simulink model "TrajectoryControl"  (R2020b)
settings: Solver=ode3  StartTime=0.0  StopTime=100.0  FixedStep=Ts  RelTol=1e-3
values from neighbouring files (symbols this model uses):
  obsx = 4    [Ejercicio1.m]    (also in Ejercicio2.m = 2.03)
  obsy = 0    [Ejercicio1.m]    (also in Ejercicio2.m = 1)
  th_0 = 0    [Ejercicio2.m]
  Ts = 100e-3    (= 0.1)    [Ejercicio1.m]    (also in Ejercicio2.m)
  x_0 = 0.02    [Ejercicio2.m]
  y_0 = 0    [Ejercicio2.m]
undefined symbols (not defined in the file or in its folder): DiscIntNeverNeededParam, sigbuilder_block
libraries: fuzblock x1, simulink x1
settings Model: Creator=patri  LastModifiedBy=Victor
settings DataIOCC: SaveOutput=off  ReturnWorkspaceOutputs=off

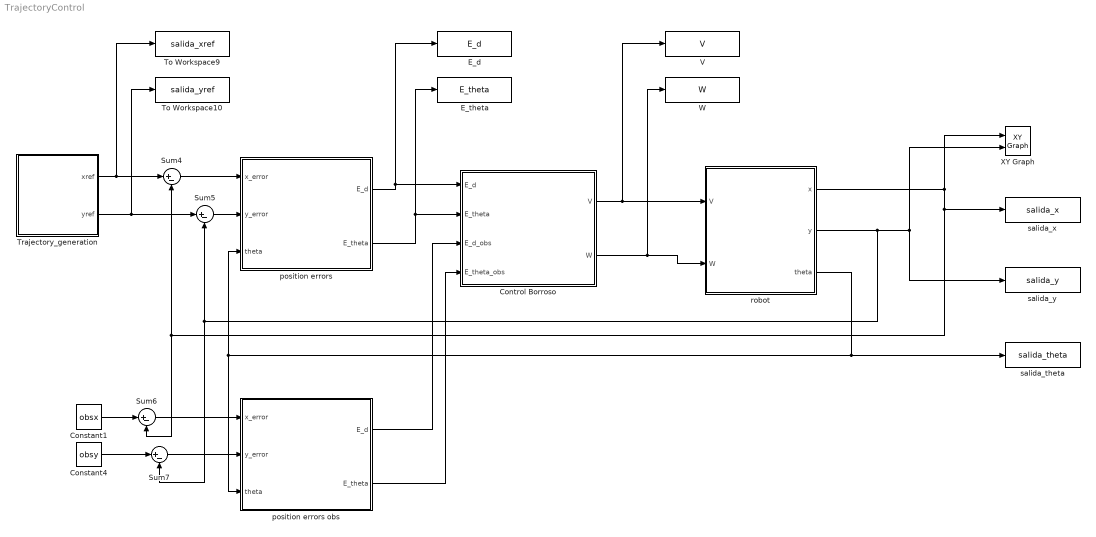
== system TrajectoryControl ==
  Constant1 : Constant  Value=obsx
  Constant4 : Constant  Value=obsy
  Control Borroso : Subsystem
  E_d : ToWorkspace  VariableName=E_d  SaveFormat=Structure With Time  SampleTime=-1
  E_theta : ToWorkspace  VariableName=E_theta  SaveFormat=Structure With Time  SampleTime=-1
  Sum{4..7} (4 alike) : Sum  Inputs=|+-
  To Workspace10 : ToWorkspace  VariableName=salida_yref  SaveFormat=Structure With Time  SampleTime=-1
  To Workspace9 : ToWorkspace  VariableName=salida_xref  SaveFormat=Structure With Time  SampleTime=-1
  Trajectory_generation : Subsystem
  V : ToWorkspace  VariableName=V  SaveFormat=Structure With Time  SampleTime=-1
  W : ToWorkspace  VariableName=W  SaveFormat=Structure With Time  SampleTime=-1
  XY Graph : simulink/Sinks/XY Graph  xmin=-10  xmax=10  ymin=-10  ymax=10  st=-1
  position errors : Subsystem
  position errors obs : Subsystem
  robot : Subsystem
  salida_theta : ToWorkspace  VariableName=salida_theta  SaveFormat=Structure With Time  SampleTime=-1
  salida_x : ToWorkspace  VariableName=salida_x  SaveFormat=Structure With Time  SampleTime=-1
  salida_y : ToWorkspace  VariableName=salida_y  SaveFormat=Structure With Time  SampleTime=-1
  wires:
  position errors obs/1(E_d) -> Control Borroso/3(E_d_obs)
  Trajectory_generation/1(xref) -> To Workspace9/1, Sum4/1
  Trajectory_generation/2(yref) -> To Workspace10/1, Sum5/1
  position errors/2(E_theta) -> Control Borroso/2(E_theta), E_theta/1
  Control Borroso/2("W ") -> robot/2(W), W/1
  Sum7/1 -> position errors obs/2(y_error)
  Constant4/1 -> Sum7/1
  position errors obs/2(E_theta) -> Control Borroso/4(E_theta_obs)
  Sum4/1 -> position errors/1(x_error)
  Constant1/1 -> Sum6/1
  Sum6/1 -> position errors obs/1(x_error)
  Sum5/1 -> position errors/2(y_error)
  robot/2(y) -> salida_y/1, XY Graph/2, Sum5/2, Sum7/2
  Control Borroso/1(V) -> V/1, robot/1(V)
  robot/1(x) -> salida_x/1, Sum4/2, Sum6/2, XY Graph/1
  position errors/1(E_d) -> Control Borroso/1("E_d "), E_d/1
  robot/3(theta) -> salida_theta/1, position errors obs/3(theta), position errors/3(theta)

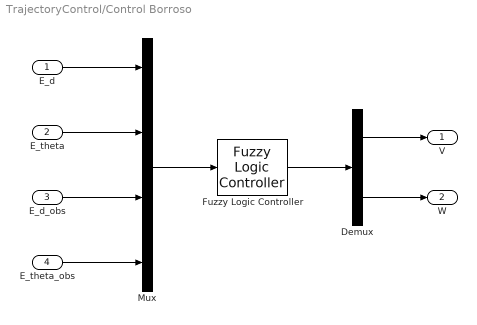
== system TrajectoryControl/Control Borroso ==
  "E_d " : Inport
  E_theta : Inport  Port=2
  E_d_obs : Inport  Port=3
  E_theta_obs : Inport  Port=4
  Demux : Demux  Outputs=2
  Fuzzy Logic Controller : fuzblock/Fuzzy Logic  Controller  FIS='ControlBorroso.fis'  OutputSampleNumber=101  DataType=double  FuzzifiedInputs=off  RuleFiringStrengths=off  RuleOutputs=off  AggregatedOutputs=off  SimulateUsing=Interpreted execution  OutOfRangeInputValueMessage=warning  NoRuleFiredMessage=warning  EmptyOutputFuzzySetMessage=warning
  Mux : Mux
  V : Outport  VectorParamsAs1DForOutWhenUnconnected=off
  "W " : Outport  Port=2  VectorParamsAs1DForOutWhenUnconnected=off
  wires:
  Mux/1 -> Fuzzy Logic Controller/1
  "E_d "/1 -> Mux/1
  Demux/1 -> V/1
  Demux/2 -> "W "/1
  E_theta/1 -> Mux/2
  E_d_obs/1 -> Mux/3
  E_theta_obs/1 -> Mux/4
  Fuzzy Logic Controller/1 -> Demux/1

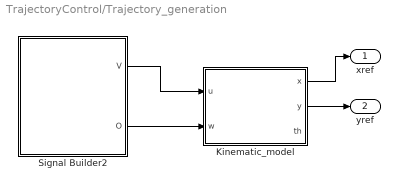
== system TrajectoryControl/Trajectory_generation ==
  Kinematic_model : Subsystem
  Signal Builder2 : Subsystem  Tag=STV Subsys  LoadFcn=sigbuilder_block('load');  StartFcn=sigbuilder_block('start');  StopFcn=sigbuilder_block('stop');  ClipboardFcn=sigbuilder_block('clipboard');  mask(Sigbuilder block){tuvar=[0:10]}
      mask help: Sigbuilder GUI
      mask init:
      | if ~strcmp(get_param(bdroot(gcbh),'SimulationStatus'),'stopped') tuvar = sigbuilder_block('maskInit'); end
      settings: CopyFcn=sigbuilder_block('copy');  DeleteFcn=sigbuilder_block('delete');  ModelCloseFcn=sigbuilder_block('modelClose');  PreSaveFcn=sigbuilder_block('preSave');  PauseFcn=sigbuilder_block('pause')  ContinueFcn=sigbuilder_block('continue')  NameChangeFcn=sigbuilder_block('namechange');  OpenFcn=sigbuilder_block('open',[60 45 534.4 467.25 ]);  CloseFcn=sigbuilder_block('close');
      mask Display: plot(0, 0, 100, 100,[2, 2, 32, 32, 2], [68, 8, 8, 68, 68],[32, 2], [38, 38], [32, 19, 2],[53, 60, 44], [32, 17, 17, 2],[16, 16, 31, 31]);txt = getActiveGroup(gcbh);text(2, 100, txt,'verticalAlignment', 'top');
  xref : Outport  VectorParamsAs1DForOutWhenUnconnected=off
  yref : Outport  Port=2  VectorParamsAs1DForOutWhenUnconnected=off
  wires:
  Kinematic_model/2(y) -> yref/1
  Kinematic_model/1(x) -> xref/1
  Signal Builder2/2(O) -> Kinematic_model/2(w)
  Signal Builder2/1(V) -> Kinematic_model/1(u)

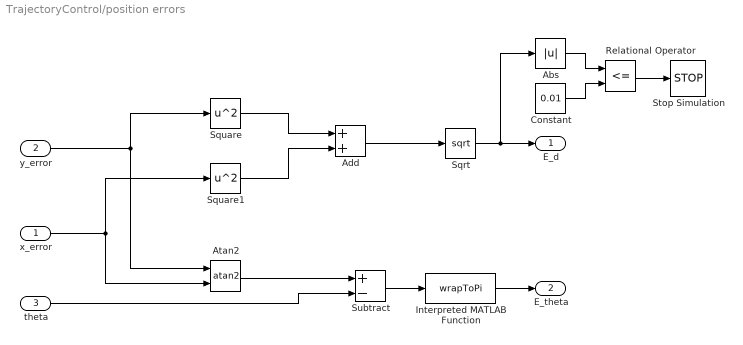
== system TrajectoryControl/position errors ==
  x_error : Inport
  y_error : Inport  Port=2
  theta : Inport  Port=3
  Abs : Abs
  Add : Sum
  Atan2 : Trigonometry  Operator=atan2
  Constant : Constant  Value=0.01
  Interpreted MATLAB Function : MATLABFcn  MATLABFcn=wrapToPi
  Relational Operator : RelationalOperator  Operator=<=  OutDataTypeStr=boolean  RndMeth=Simplest
  Sqrt : Sqrt  SaturateOnIntegerOverflow=on
  Square : Math  Operator=square  SignedPower=on  SaturateOnIntegerOverflow=on
  Square1 : Math  Operator=square  SignedPower=on  SaturateOnIntegerOverflow=on
  Stop Simulation : Stop
  Subtract : Sum  Inputs=+-  OutMin=[-3.14]  OutMax=[3.14]
  E_d : Outport  VectorParamsAs1DForOutWhenUnconnected=off
  E_theta : Outport  Port=2  OutMin=[-pi]  OutMax=[pi]  VectorParamsAs1DForOutWhenUnconnected=off
  wires:
  y_error/1 -> Atan2/1, Square/1
  x_error/1 -> Atan2/2, Square1/1
  Square/1 -> Add/1
  Square1/1 -> Add/2
  Add/1 -> Sqrt/1
  Sqrt/1 -> Abs/1, E_d/1
  Atan2/1 -> Subtract/1
  theta/1 -> Subtract/2
  Abs/1 -> Relational Operator/1
  Constant/1 -> Relational Operator/2
  Relational Operator/1 -> Stop Simulation/1
  Interpreted MATLAB Function/1 -> E_theta/1
  Subtract/1 -> Interpreted MATLAB Function/1

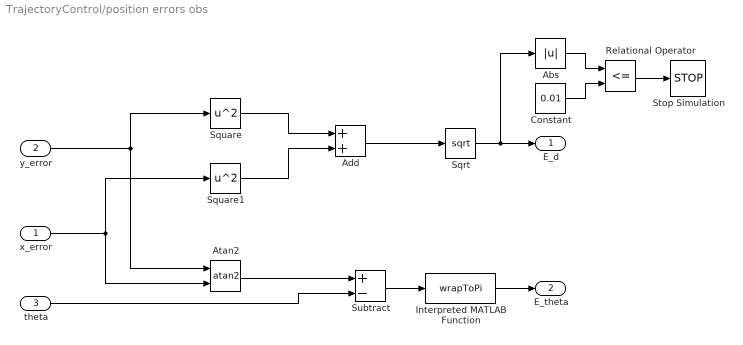
== system TrajectoryControl/position errors obs ==
  x_error : Inport
  y_error : Inport  Port=2
  theta : Inport  Port=3
  Abs : Abs
  Add : Sum
  Atan2 : Trigonometry  Operator=atan2
  Constant : Constant  Value=0.01
  Interpreted MATLAB Function : MATLABFcn  MATLABFcn=wrapToPi
  Relational Operator : RelationalOperator  Operator=<=  OutDataTypeStr=boolean  RndMeth=Simplest
  Sqrt : Sqrt  SaturateOnIntegerOverflow=on
  Square : Math  Operator=square  SignedPower=on  SaturateOnIntegerOverflow=on
  Square1 : Math  Operator=square  SignedPower=on  SaturateOnIntegerOverflow=on
  Stop Simulation : Stop
  Subtract : Sum  Inputs=+-
  E_d : Outport  VectorParamsAs1DForOutWhenUnconnected=off
  E_theta : Outport  Port=2  OutMin=[-pi]  OutMax=[pi]  VectorParamsAs1DForOutWhenUnconnected=off
  wires:
  y_error/1 -> Atan2/1, Square/1
  x_error/1 -> Atan2/2, Square1/1
  Square/1 -> Add/1
  Square1/1 -> Add/2
  Add/1 -> Sqrt/1
  Sqrt/1 -> Abs/1, E_d/1
  Atan2/1 -> Subtract/1
  theta/1 -> Subtract/2
  Abs/1 -> Relational Operator/1
  Constant/1 -> Relational Operator/2
  Relational Operator/1 -> Stop Simulation/1
  Subtract/1 -> Interpreted MATLAB Function/1
  Interpreted MATLAB Function/1 -> E_theta/1

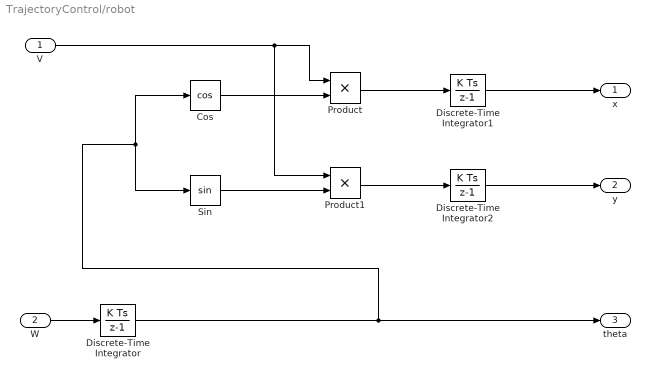
== system TrajectoryControl/robot ==
  V : Inport
  W : Inport  Port=2
  Cos : Trigonometry  Operator=cos
  Discrete-Time Integrator : DiscreteIntegrator  SampleTime=-1  ICPrevOutput=DiscIntNeverNeededParam  ICPrevScaledInput=DiscIntNeverNeededParam
  Discrete-Time Integrator1 : DiscreteIntegrator  SampleTime=-1  ICPrevOutput=DiscIntNeverNeededParam  ICPrevScaledInput=DiscIntNeverNeededParam
  Discrete-Time Integrator2 : DiscreteIntegrator  SampleTime=-1  ICPrevOutput=DiscIntNeverNeededParam  ICPrevScaledInput=DiscIntNeverNeededParam
  Product : Product
  Product1 : Product
  Sin : Trigonometry
  x : Outport  VectorParamsAs1DForOutWhenUnconnected=off
  y : Outport  Port=2  VectorParamsAs1DForOutWhenUnconnected=off
  theta : Outport  Port=3  VectorParamsAs1DForOutWhenUnconnected=off
  wires:
  Sin/1 -> Product1/2
  Product1/1 -> Discrete-Time Integrator2/1
  Product/1 -> Discrete-Time Integrator1/1
  Discrete-Time Integrator2/1 -> y/1
  V/1 -> Product1/1, Product/1
  Discrete-Time Integrator1/1 -> x/1
  Discrete-Time Integrator/1 -> theta/1, Sin/1, Cos/1
  W/1 -> Discrete-Time Integrator/1
  Cos/1 -> Product/2

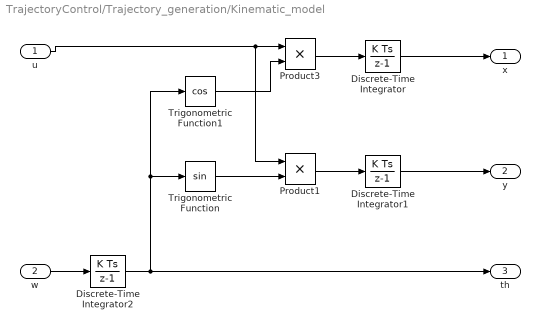
== system TrajectoryControl/Trajectory_generation/Kinematic_model ==
  u : Inport
  w : Inport  Port=2
  Discrete-Time Integrator : DiscreteIntegrator  InitialCondition=x_0  SampleTime=Ts  ICPrevOutput=DiscIntNeverNeededParam  ICPrevScaledInput=DiscIntNeverNeededParam
  Discrete-Time Integrator1 : DiscreteIntegrator  InitialCondition=y_0  SampleTime=Ts  ICPrevOutput=DiscIntNeverNeededParam  ICPrevScaledInput=DiscIntNeverNeededParam
  Discrete-Time Integrator2 : DiscreteIntegrator  InitialCondition=th_0  SampleTime=Ts  ICPrevOutput=DiscIntNeverNeededParam  ICPrevScaledInput=DiscIntNeverNeededParam
  Product1 : Product
  Product3 : Product
  Trigonometric Function : Trigonometry
  Trigonometric Function1 : Trigonometry  Operator=cos
  x : Outport  VectorParamsAs1DForOutWhenUnconnected=off
  y : Outport  Port=2  VectorParamsAs1DForOutWhenUnconnected=off
  th : Outport  Port=3  VectorParamsAs1DForOutWhenUnconnected=off
  wires:
  Discrete-Time Integrator/1 -> x/1
  Discrete-Time Integrator1/1 -> y/1
  Trigonometric Function1/1 -> Product3/2
  u/1 -> Product3/1, Product1/1
  Trigonometric Function/1 -> Product1/2
  w/1 -> Discrete-Time Integrator2/1
  Product3/1 -> Discrete-Time Integrator/1
  Product1/1 -> Discrete-Time Integrator1/1
  Discrete-Time Integrator2/1 -> th/1, Trigonometric Function/1, Trigonometric Function1/1

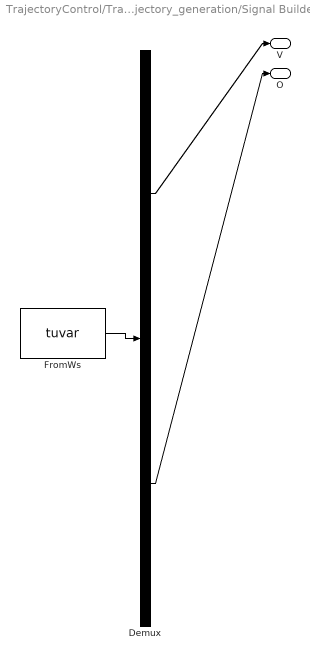
== system TrajectoryControl/Trajectory_generation/Signal Builder2 ==
  Demux : Demux  Tag=STV Demux  Outputs=2
      settings: DisplayOption=none
  FromWs : FromWorkspace  Tag=STV FromWs  VariableName=tuvar
      SigBuilderData=|
      | common.afterFinalStr = 'Extrapolate'
      | common.sampleTime = '0'
      | dataSet.timeRange = [0 115]
      | dataSet.name = 'Group 1'
      | sbobj.Groups.Name = 'Group 1'
      | sbobj.Groups.Signals(1).Name = 'V'
      | sbobj.Groups.Signals(1).XData = [0 87 87 115]
      | sbobj.Groups.Signals(1).YData = [0.25 0.25 0 0]
      | sbobj.Groups.Signals(2).Name = 'O'
      | sbobj.Groups.Signals(2).XData = [0 12 12 30.849 30.849 55.981 55.981 74.83 74.83 99.962 115]
      | sbobj.Groups.Signals(2).YData = [0 0 0.25 0.25 -0.25 -0.25 0.25 0.25 0 0 0]
      | sbobj.Groups.TimeRange = [0 115]
  V : Outport  Tag=STV Outport  VectorParamsAs1DForOutWhenUnconnected=off
  O : Outport  Tag=STV Outport  Port=2  VectorParamsAs1DForOutWhenUnconnected=off
  wires:
  Demux/2 -> O/1
  Demux/1 -> V/1
  FromWs/1 -> Demux/1
